simulink model "gazebo_imu"  (R2019b)
settings: Solver=VariableStepAuto  StartTime=0.0  StopTime=10.0  RelTol=1e-3
libraries: robotgazebolib x2, robotcorelib x1
settings Model: Creator=darrahts  LastModifiedBy=darrahts

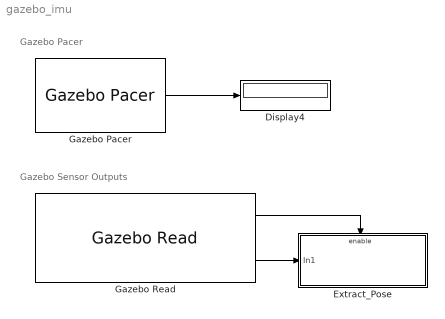
== system gazebo_imu ==
  note: Gazebo Pacer
  note: Gazebo Sensor Outputs
  Display4 : Display
  Extract_Pose : Subsystem
  Gazebo Pacer : robotgazebolib/Gazebo Pacer  ResetBehavior=Reset Gazebo simulation time and scene  SampleTime=0.01
      settings: SourceProductName=Robotics System Toolbox  SourceProductBaseCode=RO
  Gazebo Read : robotgazebolib/Gazebo Read  topicSource=From Gazebo  topic=/gazebo/ground_truth/world_pose/iris/base_link  messageType=gazebo_msgs/Pose  sampleTime=.01
      settings: SourceProductName=Robotics System Toolbox  SourceProductBaseCode=RO
  wires:
  Gazebo Pacer/1 -> Display4/1
  Gazebo Read/1 -> Extract_Pose/Enable
  Gazebo Read/2 -> Extract_Pose/1(In1)

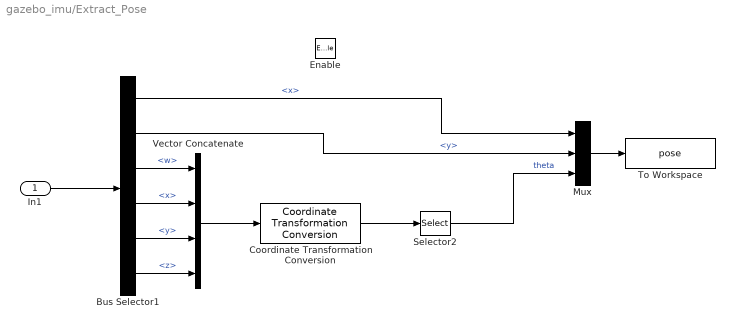
== system gazebo_imu/Extract_Pose ==
  In1 : Inport
  Enable : EnablePort
  Bus Selector1 : BusSelector  OutputSignals=position.x,position.y,orientation.w,orientation.x,orientation.y,orientation.z
  Coordinate Transformation Conversion : robotcorelib/Coordinate Transformation Conversion  InputRepresentation=Quaternion  InputEulerSequence=ZYX  ShowTrVecInputPort=on  OutputRepresentation=Euler Angles  OutputEulerSequence=ZYX  ShowTrVecOutputPort=on  SimulateUsing=Interpreted execution
      settings: SourceProductBaseCode=RO
  Mux : Mux  Inputs=3
  Selector2 : Selector  InputPortWidth=3  IndexOptions=Index vector (dialog)  Indices=1  OutputSizes=1
  To Workspace : ToWorkspace  VariableName=pose  SaveFormat=Timeseries  SampleTime=-1
  Vector Concatenate : Concatenate  NumInputs=4
  wires:
  Vector Concatenate/1 -> Coordinate Transformation Conversion/1
  Coordinate Transformation Conversion/1 -> Selector2/1
  Selector2/1 -> Mux/3  "theta"
  Bus Selector1/6 -> Vector Concatenate/4  "<z>"
  Bus Selector1/4 -> Vector Concatenate/2  "<x>"
  Bus Selector1/3 -> Vector Concatenate/1  "<w>"
  Bus Selector1/5 -> Vector Concatenate/3  "<y>"
  In1/1 -> Bus Selector1/1
  Bus Selector1/1 -> Mux/1  "<x>"
  Bus Selector1/2 -> Mux/2  "<y>"
  Mux/1 -> To Workspace/1
